simulink model "SF048A_TqLoa"  (R2013b)
settings: Solver=FixedStepDiscrete  SolverMode=SingleTasking  StartTime=0.0  StopTime=1  FixedStep=0.002  RelTol=1e-3
values from neighbouring files (symbols this model uses):
  ARCHGLBPRM_2MILLISEC_SEC_F32 = DataDict.Constant    [SF048A_TqLoa_DataDict.m]
  ARCHGLBPRM_PIOVER180_ULS_F32 = DataDict.Constant    [SF048A_TqLoa_DataDict.m]
  GRVYTLCON_MTRPERSECSQD_F32 = DataDict.Constant    [SF048A_TqLoa_DataDict.m]
  HWAUTHYMIN_ULS_F32 = DataDict.Constant    [SF048A_TqLoa_DataDict.m]
  MTRPERSECOVERKPH_MTRPERSECPERKPH_F32 = DataDict.Constant    [SF048A_TqLoa_DataDict.m]
  TqLoaDrvrTqNom = DataDict.Calibration    [SF048A_TqLoa_DataDict.m]
  TqLoaMotTqCmdLim = DataDict.Calibration    [SF048A_TqLoa_DataDict.m]
  TqLoaMotVelAndTqBasdScaFacMax = DataDict.Calibration    [SF048A_TqLoa_DataDict.m]
  TqLoaMotVelAndTqBasdScaFacMin = DataDict.Calibration    [SF048A_TqLoa_DataDict.m]
  TqLoaMotVelMgnThd = DataDict.Calibration    [SF048A_TqLoa_DataDict.m]
  TqLoaTqCmdMgnThd = DataDict.Calibration    [SF048A_TqLoa_DataDict.m]
  TqLoaVehSteerRat = DataDict.Calibration    [SF048A_TqLoa_DataDict.m]
  TqLoaVehUnderSteerGrdt = DataDict.Calibration    [SF048A_TqLoa_DataDict.m]
  TqLoaVehWhlBas = DataDict.Calibration    [SF048A_TqLoa_DataDict.m]
libraries: NxtrLim x8, FloatToFixd x5, FixdToFloat x4, LnrIntrpn x3, simulink x2, Fil x2, BilnrIntrpnCmnX x1
(part 1 of 2)
Description:
  | This function uses vehicle speed and HW position to generate a temporary position-based assist command.
  | This command is further scaled down based on vehicle speed, motor velocity and measured lateral
  | acceleration, to produce a final TLOA command.
settings Model: Creator=HZ69BY  LastModifiedBy=XZB1DB
settings Model: ModifiedHistory=|
  | Change Log:
  | Rev: 001
  | Date: 01Feb2015
  | Change Control #:
  | DRW:
  | Description:
  | - Initial Release
  | 
  | Rev: 002
  | Date: 05May2015
  | Change Request:  EA3#1132
  | Description:
  | - Removed Saturation from SF48A_TrqLOA_v002/TrqLOA/TrqLOA/Scaling/MtrVelBasedScaling/Torque-Velocity Based
  | - Added Saturation to SF48A_TrqLOA_v002/TrqLOA/TrqLOA/Scaling/VehicleSpeedBasedScaling
  | - Saturation limits set as constants from data dictionary
  | - Low-pass filter updated as per EA3 Simulink library (SF48A_TrqLOA_v002/TrqLOA/TrqLOA/Scaling/LatAccBasedScaling)
  | - Data Dictionary Changes:
  |    - t2_TrqLOA_DiffGainY_Uls_u1p15 name, table size, default value updated.
  |    - t_TrqLOA_DiffGainX_G_u2p14 default value updated
  |    - Changed range for k_TrqLOA_LimOutput_MtrNm_f32 & TrqLOACmd_MtrNm_f32
  |    - Added Constants d_TrqLOA_MinScale_Uls_f32 & d_TrqLOA_MaxScale_Uls_f32
  |    - Initial value of MotAgLoaMtgtnEn_Cnt_lgc changed to 0
  |    - Increased length/size of t_TrqLOA_X_Kph, t_TrqLOA_LatAccGain_Y_MtrNmpG, t_TrqLOA_TempTrqCmdSatYTbl_MtrNm
settings SolverCC: AutoInsertRateTranBlk=on  InsertRTBMode=Always
settings DataIOCC: LimitDataPoints=off  SaveFormat=Structure  ReturnWorkspaceOutputs=on
settings OptimizationCC: BlockReduction=off  InlineParams=on  ZeroExternalMemoryAtStartup=off  ZeroInternalMemoryAtStartup=off  OptimizeModelRefInitCode=on  LifeSpan=1
settings DebuggingCC: SignalInfNanChecking=error  SignalRangeChecking=warning  UnderspecifiedInitializationDetection=Simplified  SolverPrmCheckMsg=error  InheritedTsInSrcMsg=error  DiscreteInheritContinuousMsg=error  SingleTaskRateTransMsg=error  TasksWithSamePriorityMsg=error  SigSpecEnsureSampleTimeMsg=error  CheckMatrixSingularityMsg=error  ParameterUnderflowMsg=error  ParameterPrecisionLossMsg=error  ParameterTunabilityLossMsg=error  FixptConstUnderflowMsg=warning  FixptConstOverflowMsg=warning  VectorMatrixConversionMsg=error  SignalLabelMismatchMsg=error  UnconnectedInputMsg=error  UnconnectedOutputMsg=error  UnconnectedLineMsg=error  SFcnCompatibilityMsg=error  UniqueDataStoreMsg=warning  BusObjectLabelMismatch=error  RootOutportRequireBusObject=error  AssertControl=DisableAll  ModelReferenceIOMsg=error  ModelReferenceVersionMismatchMessage=warning  ModelReferenceIOMismatchMessage=error  ModelReferenceCSMismatchMessage=warning  ModelReferenceDataLoggingMessage=error  StateNameClashWarn=warning  StrictBusMsg=ErrorOnBusTreatedAsVector  NonBusSignalsTreatedAsBus=error  SFUnexpectedBacktrackingDiag=error  SFInvalidInputDataAccessInChartInitDiag=error  SFNoUnconditionalDefaultTransitionDiag=error  SFTransitionOutsideNaturalParentDiag=error  SFUnconditionalTransitionShadowingDiag=error  SFUndirectedBroadcastEventsDiag=error
settings ModelReferenceCC: ModelReferenceNumInstancesAllowed=Single
settings RTWCC: SystemTargetFile=autosar.tlc  GenCodeOnly=on  TemplateMakefile=ert_default_tmf  Description=AUTOSAR  GenerateReport=on  ProcessScript=autosar_make_rtw_hook  LaunchReport=on
settings CodeAppCC: GenerateComments=off  IgnoreCustomStorageClasses=off  CustomSymbolStrType=$N$R$M  CustomSymbolStrBlkIO=$N$M  SimulinkBlockComments=off
settings STFCustomTargetCC: ParMdlRefBuildCompliant=on  CompOptLevelCompliant=on  IncludeMdlTerminateFcn=off  CombineOutputUpdateFcns=on  SuppressErrorStatus=on  ERTFirstTimeCompliant=on  ERTCustomFileBanners=on  SupportNonFinite=off  SupportComplex=off  SupportContinuousTime=off  SupportNonInlinedSFcns=off  MATLABClassNameForMDSCustomization=Simulink.SoftwareTarget.ERTCustomization  AutosarCompliant=on  GRTInterface=off  SystemTargetFile=autosar.tlc
settings ERTTargetCC: CodeReplacementLibrary=ANSI_C  ConcurrentExecutionCompliant=off  IncludeMdlTerminateFcn=off  SuppressErrorStatus=on  SupportNonFinite=off  SupportComplex=off  ModelStepFunctionPrototypeControlCompliant=off  CPPClassGenCompliant=off  AutosarCompliant=on  InlinedParameterPlacement=NonHierarchical  ERTCustomFileTemplate=example_file_process.tlc  EnableUserReplacementTypes=on

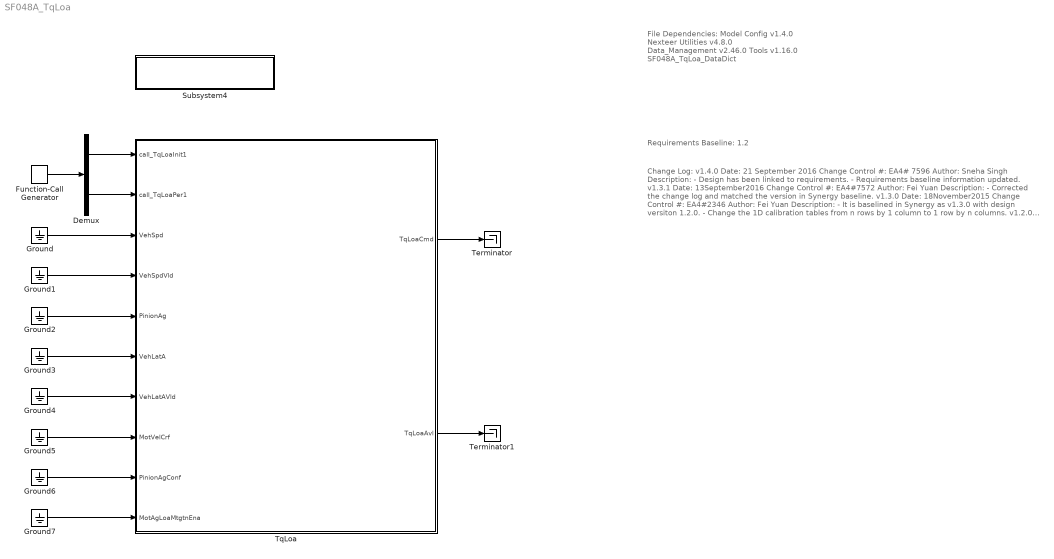
== system SF048A_TqLoa ==
  note: File Dependencies:
      |
      | Model Config v1.4.0
      | Nexteer Utilities v4.8.0
      | Data_Management v2.46.0
      | Tools v1.16.0
      | SF048A_TqLoa_DataDict
  note: Change Log:
      |
      | v1.4.0
      | Date: 21 September 2016
      | Change Control #: EA4# 7596
      | Author: Sneha Singh
      | Description:
      | - Design has been linked to requirements.
      | - Requirements baseline information updated.
      |
      | v1.3.1
      | Date: 13September2016
      | Change Control #: EA4#7572
      | Author: Fei Yuan
      | Description:
      | - Corrected the change log and matched the version in Synergy baseline.
      |
      | v1.3.0
      | Date: 18November2015
      | Change Control #: EA4#2346
      | Author: Fei Yuan
      | Description:
      | - It is baselined in Synergy as v1.3.0 with design versiton 1.2.0.
      | - Change the 1D calibration tables from n rows by 1 column to 1 row by n
      |   columns.
      |
      | v1.2.0
      | Date: 01September2015
      | Change Control #: EA4#1010
      | DRW: P.Lefler
      | Description:
      | - It is baselined in Synergy as v1.2.0 with design version 1.1.0.
      |
      |
      | v1.1.0
      | Date: 01September2015
      | Change Control #: EA4#1010
      | DRW: P. Lefler
      | Description:
      | - Fixed reversed order of constants in static limit blocks.
      | - Removed extra write to a display variable.
      | - Changed inputs from HwAg and HwAuthy to PinionAgConf and PinionAg
      |
      |
      | v1.0.0
      | Date: 30July2015
      | Change Control #: EA4#1010
      | DRW: P. Lefler
      | Description:
      | - Initial Release
  note: Requirements Baseline: 1.2
  Demux : Demux  Outputs=2
  Function-Call Generator : simulink/Ports & Subsystems/Function-Call Generator  sample_time=0.002  numberOfIterations=1
  Ground{,1..7} (8 alike) : Ground
  Subsystem4 : Subsystem  Description=|  mask(Copyright Information){none=on}
      | Copyright info block.                                               
      |                                                                     
      | Place copyright information at the top of every subsystem in design.
      mask prompts: none "No parameters"
      mask help: Place copyright information at the top of every subsystem in design.
      mask Display:
      | NxtrConf = 'Nexteer Confidential';
      | 
      | sys = bdroot; %handle for the current model ("system")
      | first = get_param(sys,'Created');
      | first = first(end-3:end);  %year is last four digits
      | 
      | last = get_param(sys,'LastModifiedDate');
      | if isempty(last)
      |     last = datestr(now,'yyyy');
      | else
      |     last = last(end-3:end);
      | end
      | 
      | if strcmp(first,last)
      |     fprintf('%s\nCopyright  %s Nexteer',NxtrConf,first);
      | else
      |     fprintf('%s\n%s%s-%s Nexteer',NxtrConf,char(169),first,last);
      | end
  Terminator : Terminator
  Terminator1 : Terminator
  TqLoa : Subsystem
  wires:
  TqLoa/1(TqLoaCmd) -> Terminator/1
  TqLoa/2(TqLoaAvl) -> Terminator1/1
  Ground7/1 -> TqLoa/10(MotAgLoaMtgtnEna)
  Ground6/1 -> TqLoa/9(PinionAgConf)
  Demux/1 -> TqLoa/1(call_TqLoaInit1)
  Demux/2 -> TqLoa/2(call_TqLoaPer1)
  Function-Call Generator/1 -> Demux/1
  Ground4/1 -> TqLoa/7(VehLatAVld)
  Ground2/1 -> TqLoa/5(PinionAg)
  Ground/1 -> TqLoa/3(VehSpd)
  Ground1/1 -> TqLoa/4(VehSpdVld)
  Ground3/1 -> TqLoa/6(VehLatA)
  Ground5/1 -> TqLoa/8(MotVelCrf)

== system SF048A_TqLoa/Subsystem4 ==

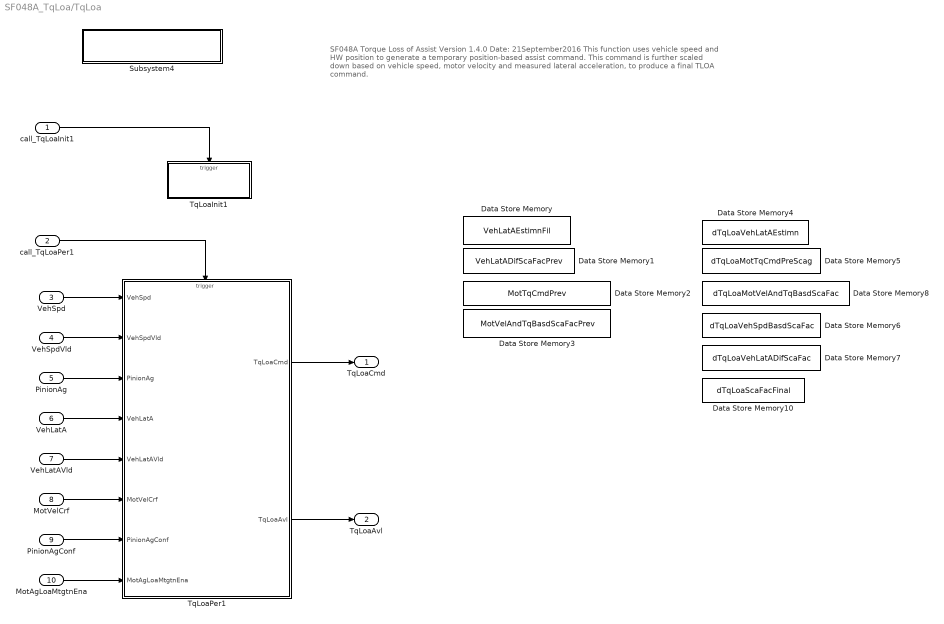
== system SF048A_TqLoa/TqLoa ==
  note: SF048A Torque Loss of Assist
      | Version 1.4.0			Date: 21September2016
      | This function uses vehicle speed and HW position to generate a temporary position-based assist command.
      | This command is further scaled down based on vehicle speed, motor velocity and measured lateral
      | acceleration, to produce a final TLOA command.
  call_TqLoaInit1 : Inport
  call_TqLoaPer1 : Inport  Port=2
  VehSpd : Inport  RequirementInfo="{'linktype_rmi_doors' '0000ba57 (/E-STEER Core/SubSystem Specifications/Application Functions/SF048A Torque Sensor LOA)' '#SF048A_6' 'true' 'REQ:  SF048A_6' '' } %GIDa_a3883147_9782_4e4b_8e21_1803a965b4c0"  Port=3
  VehSpdVld : Inport  RequirementInfo="{'linktype_rmi_doors' '0000ba57 (/E-STEER Core/SubSystem Specifications/Application Functions/SF048A Torque Sensor LOA)' '#SF048A_6' 'true' 'REQ:  SF048A_6' '' } %GIDa_02708a8b_8017_404a_990b_357237815eff"  Port=4
  PinionAg : Inport  RequirementInfo="{'linktype_rmi_doors' '0000ba57 (/E-STEER Core/SubSystem Specifications/Application Functions/SF048A Torque Sensor LOA)' '#SF048A_7' 'true' 'REQ:  SF048A_7' '' } %GIDa_9e569ae1_e816_4a3a_b96f_f5710bee6e9e"  Port=5
  VehLatA : Inport  RequirementInfo="{'linktype_rmi_doors' '0000ba57 (/E-STEER Core/SubSystem Specifications/Application Functions/SF048A Torque Sensor LOA)' '#SF048A_40' 'true' 'REQ:  SF048A_40' '' } %GIDa_13b7e215_ca06_42b4_96ce_87e09b7122fe"  Port=6
  VehLatAVld : Inport  RequirementInfo="{'linktype_rmi_doors' '0000ba57 (/E-STEER Core/SubSystem Specifications/Application Functions/SF048A Torque Sensor LOA)' '#SF048A_41' 'true' 'REQ:  SF048A_41' '' } %GIDa_2dd0dbe9_8486_4322_8285_2c1192106a5d"  Port=7
  MotVelCrf : Inport  RequirementInfo="{'linktype_rmi_doors' '0000ba57 (/E-STEER Core/SubSystem Specifications/Application Functions/SF048A Torque Sensor LOA)' '#SF048A_42' 'true' 'REQ:  SF048A_42' '' } %GIDa_5a1973eb_7739_48b8_9cc6_d351e8423a12"  Port=8
  PinionAgConf : Inport  RequirementInfo="{'linktype_rmi_doors' '0000ba57 (/E-STEER Core/SubSystem Specifications/Application Functions/SF048A Torque Sensor LOA)' '#SF048A_8' 'true' 'REQ:  SF048A_8' '' } %GIDa_aa7a9f1f_eb7f_4301_85f9_898c0a77cdeb"  Port=9
  MotAgLoaMtgtnEna : Inport  RequirementInfo="{'linktype_rmi_doors' '0000ba57 (/E-STEER Core/SubSystem Specifications/Application Functions/SF048A Torque Sensor LOA)' '#SF048A_43' 'true' 'REQ:  SF048A_43' '' } %GIDa_2270dc32_128a_4873_b3c1_ebcb33cb1a8b"  Port=10
  Data Store Memory : DataStoreMemory  DataStoreName=VehLatAEstimnFil  InitialValue=[]  StateMustResolveToSignalObject=on
  Data Store Memory1 : DataStoreMemory  DataStoreName=VehLatADifScaFacPrev  StateMustResolveToSignalObject=on
  Data Store Memory10 : DataStoreMemory  DataStoreName=dTqLoaScaFacFinal  ReadBeforeWriteMsg=warning  WriteAfterWriteMsg=warning  WriteAfterReadMsg=warning  StateMustResolveToSignalObject=on
  Data Store Memory2 : DataStoreMemory  DataStoreName=MotTqCmdPrev  StateMustResolveToSignalObject=on
  Data Store Memory3 : DataStoreMemory  DataStoreName=MotVelAndTqBasdScaFacPrev  StateMustResolveToSignalObject=on
  Data Store Memory4 : DataStoreMemory  DataStoreName=dTqLoaVehLatAEstimn  ReadBeforeWriteMsg=warning  WriteAfterWriteMsg=warning  WriteAfterReadMsg=warning  StateMustResolveToSignalObject=on
  Data Store Memory5 : DataStoreMemory  DataStoreName=dTqLoaMotTqCmdPreScag  ReadBeforeWriteMsg=warning  WriteAfterWriteMsg=warning  WriteAfterReadMsg=warning  StateMustResolveToSignalObject=on
  Data Store Memory6 : DataStoreMemory  DataStoreName=dTqLoaVehSpdBasdScaFac  ReadBeforeWriteMsg=warning  WriteAfterWriteMsg=warning  WriteAfterReadMsg=warning  StateMustResolveToSignalObject=on
  Data Store Memory7 : DataStoreMemory  DataStoreName=dTqLoaVehLatADifScaFac  ReadBeforeWriteMsg=warning  WriteAfterWriteMsg=warning  WriteAfterReadMsg=warning  StateMustResolveToSignalObject=on
  Data Store Memory8 : DataStoreMemory  DataStoreName=dTqLoaMotVelAndTqBasdScaFac  ReadBeforeWriteMsg=warning  WriteAfterWriteMsg=warning  WriteAfterReadMsg=warning  StateMustResolveToSignalObject=on
  Subsystem4 : Subsystem  Description=|  mask(Copyright Information){none=on}
      | Copyright info block.                                               
      |                                                                     
      | Place copyright information at the top of every subsystem in design.
      mask prompts: none "No parameters"
      mask help: Place copyright information at the top of every subsystem in design.
      mask Display:
      | NxtrConf = 'Nexteer Confidential';
      | 
      | sys = bdroot; %handle for the current model ("system")
      | first = get_param(sys,'Created');
      | first = first(end-3:end);  %year is last four digits
      | 
      | last = get_param(sys,'LastModifiedDate');
      | if isempty(last)
      |     last = datestr(now,'yyyy');
      | else
      |     last = last(end-3:end);
      | end
      | 
      | if strcmp(first,last)
      |     fprintf('%s\nCopyright  %s Nexteer',NxtrConf,first);
      | else
      |     fprintf('%s\n%s%s-%s Nexteer',NxtrConf,char(169),first,last);
      | end
  TqLoaInit1 : Subsystem
  TqLoaPer1 : Subsystem
  TqLoaCmd : Outport  RequirementInfo="{'linktype_rmi_doors' '0000ba57 (/E-STEER Core/SubSystem Specifications/Application Functions/SF048A Torque Sensor LOA)' '#SF048A_10' 'true' 'REQ:  SF048A_10' '' } %GIDa_df82e166_2ee0_4c30_8d9b_00a7e29d6193"
  TqLoaAvl : Outport  RequirementInfo="{'linktype_rmi_doors' '0000ba57 (/E-STEER Core/SubSystem Specifications/Application Functions/SF048A Torque Sensor LOA)' '#SF048A_44' 'true' 'REQ:  SF048A_44' '' } %GIDa_bf8a2443_6d8b_4475_a369_59109990c7ac"  Port=2
  wires:
  MotAgLoaMtgtnEna/1 -> TqLoaPer1/8(MotAgLoaMtgtnEna)
  MotVelCrf/1 -> TqLoaPer1/6(MotVelCrf)
  VehLatAVld/1 -> TqLoaPer1/5(VehLatAVld)
  PinionAg/1 -> TqLoaPer1/3(PinionAg)
  VehSpdVld/1 -> TqLoaPer1/2(VehSpdVld)
  VehLatA/1 -> TqLoaPer1/4(VehLatA)
  PinionAgConf/1 -> TqLoaPer1/7(PinionAgConf)
  VehSpd/1 -> TqLoaPer1/1(VehSpd)
  TqLoaPer1/1(TqLoaCmd) -> TqLoaCmd/1
  TqLoaPer1/2(TqLoaAvl) -> TqLoaAvl/1
  call_TqLoaPer1/1 -> TqLoaPer1/Trigger
  call_TqLoaInit1/1 -> TqLoaInit1/Trigger

== system SF048A_TqLoa/TqLoa/Subsystem4 ==

== system SF048A_TqLoa/TqLoa/TqLoaInit1 ==
  Function : TriggerPort  TriggerType=function-call  PortDimensions=1
  FilLpInit : Fil/FilLpInit  Ic=0  Ts=ARCHGLBPRM_2MILLISEC_SEC_F32  Freq=TqLoaVehLatAEstimnFilFrq  StVar=VehLatAEstimnFil
  Subsystem4 : Subsystem  Description=|  mask(Copyright Information){none=on}
      | Copyright info block.                                               
      |                                                                     
      | Place copyright information at the top of every subsystem in design.
      mask prompts: none "No parameters"
      mask help: Place copyright information at the top of every subsystem in design.
      mask Display:
      | NxtrConf = 'Nexteer Confidential';
      | 
      | sys = bdroot; %handle for the current model ("system")
      | first = get_param(sys,'Created');
      | first = first(end-3:end);  %year is last four digits
      | 
      | last = get_param(sys,'LastModifiedDate');
      | if isempty(last)
      |     last = datestr(now,'yyyy');
      | else
      |     last = last(end-3:end);
      | end
      | 
      | if strcmp(first,last)
      |     fprintf('%s\nCopyright  %s Nexteer',NxtrConf,first);
      | else
      |     fprintf('%s\n%s%s-%s Nexteer',NxtrConf,char(169),first,last);
      | end

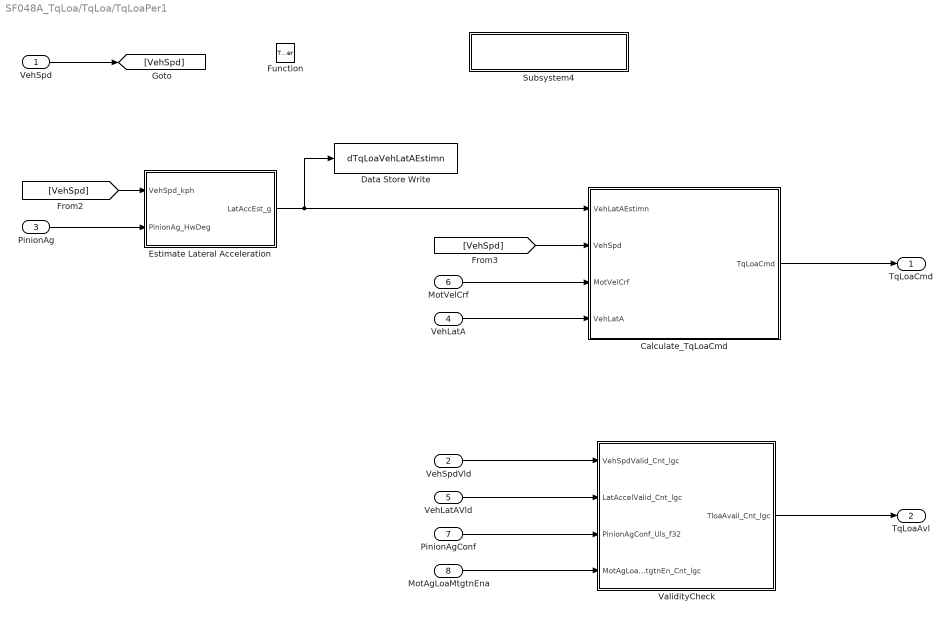
== system SF048A_TqLoa/TqLoa/TqLoaPer1 ==
  VehSpd : Inport
  VehSpdVld : Inport  Port=2
  PinionAg : Inport  Port=3
  VehLatA : Inport  Port=4
  VehLatAVld : Inport  Port=5
  MotVelCrf : Inport  Port=6
  PinionAgConf : Inport  Port=7
  MotAgLoaMtgtnEna : Inport  Port=8
  Function : TriggerPort  TriggerType=function-call  PortDimensions=1
  Calculate_TqLoaCmd : Subsystem
  Data Store Write : DataStoreWrite  DataStoreName=dTqLoaVehLatAEstimn
  Estimate Lateral Acceleration : Subsystem  RequirementInfo="{'linktype_rmi_doors' '0000ba57 (/E-STEER Core/SubSystem Specifications/Application Functions/SF048A Torque Sensor LOA)' '#SF048A_57' 'true' 'REQ:  SF048A_57' '' } %GIDa_a7e7015c_6445_44b2_86c9_655a6d6cfbb8"
  Subsystem4 : Subsystem  Description=|  mask(Copyright Information){none=on}
      | Copyright info block.                                               
      |                                                                     
      | Place copyright information at the top of every subsystem in design.
      mask prompts: none "No parameters"
      mask help: Place copyright information at the top of every subsystem in design.
      mask Display:
      | NxtrConf = 'Nexteer Confidential';
      | 
      | sys = bdroot; %handle for the current model ("system")
      | first = get_param(sys,'Created');
      | first = first(end-3:end);  %year is last four digits
      | 
      | last = get_param(sys,'LastModifiedDate');
      | if isempty(last)
      |     last = datestr(now,'yyyy');
      | else
      |     last = last(end-3:end);
      | end
      | 
      | if strcmp(first,last)
      |     fprintf('%s\nCopyright  %s Nexteer',NxtrConf,first);
      | else
      |     fprintf('%s\n%s%s-%s Nexteer',NxtrConf,char(169),first,last);
      | end
  ValidityCheck : Subsystem
  TqLoaCmd : Outport
  TqLoaAvl : Outport  Port=2
  wires:
  Estimate Lateral Acceleration/1(LatAccEst_g) -> Data Store Write/1, Calculate_TqLoaCmd/1(VehLatAEstimn)
  [VehSpd] -> Estimate Lateral Acceleration/1(VehSpd_kph)
  ValidityCheck/1(TloaAvail_Cnt_lgc) -> TqLoaAvl/1
  VehSpd/1 -> [VehSpd]
  VehSpdVld/1 -> ValidityCheck/1(VehSpdValid_Cnt_lgc)
  MotAgLoaMtgtnEna/1 -> ValidityCheck/4(MotAgLoaMtgtnEn_Cnt_lgc)
  PinionAgConf/1 -> ValidityCheck/3(PinionAgConf_Uls_f32)
  VehLatAVld/1 -> ValidityCheck/2(LatAccelValid_Cnt_lgc)
  PinionAg/1 -> Estimate Lateral Acceleration/2(PinionAg_HwDeg)
  [VehSpd] -> Calculate_TqLoaCmd/2(VehSpd)
  MotVelCrf/1 -> Calculate_TqLoaCmd/3(MotVelCrf)
  VehLatA/1 -> Calculate_TqLoaCmd/4(VehLatA)
  Calculate_TqLoaCmd/1(TqLoaCmd) -> TqLoaCmd/1

== system SF048A_TqLoa/TqLoa/TqLoaInit1/Subsystem4 ==

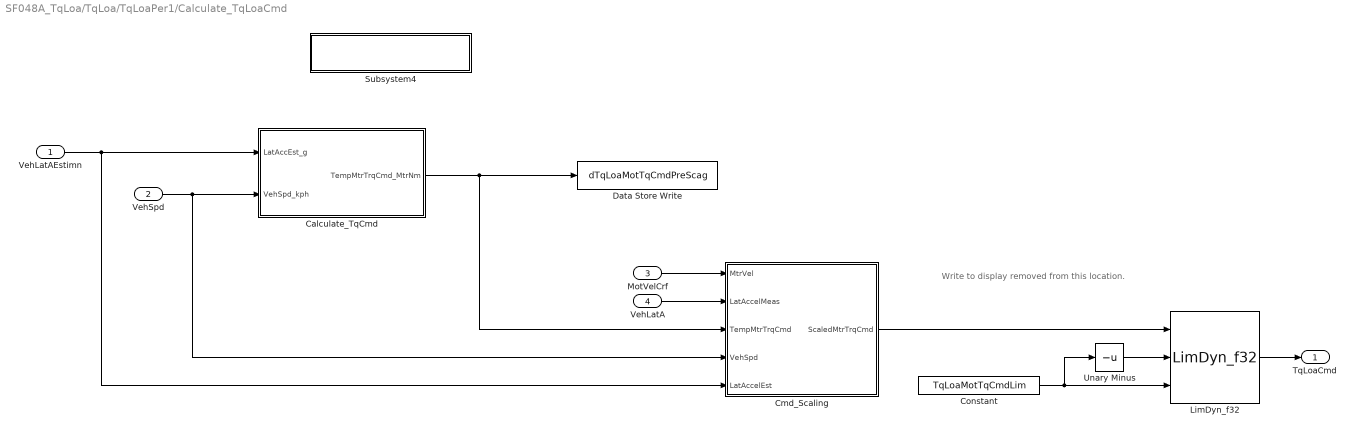
== system SF048A_TqLoa/TqLoa/TqLoaPer1/Calculate_TqLoaCmd ==
  note: Write to display removed from this location.
  VehLatAEstimn : Inport
  VehSpd : Inport  Port=2
  MotVelCrf : Inport  Port=3
  VehLatA : Inport  Port=4
  Calculate_TqCmd : Subsystem
  Cmd_Scaling : Subsystem
  Constant : Constant  RequirementInfo="{'linktype_rmi_doors' '0000ba57 (/E-STEER Core/SubSystem Specifications/Application Functions/SF048A Torque Sensor LOA)' '#SF048A_83' 'true' 'REQ:  SF048A_83' '' } %GIDa_345a0c70_3a23_42e4_82c5_17cc6df77ff3"  Value=TqLoaMotTqCmdLim
  Data Store Write : DataStoreWrite  DataStoreName=dTqLoaMotTqCmdPreScag
  LimDyn_f32 : NxtrLim/LimDyn_f32  RequirementInfo="{'linktype_rmi_doors' '0000ba57 (/E-STEER Core/SubSystem Specifications/Application Functions/SF048A Torque Sensor LOA)' '#SF048A_83' 'true' 'REQ:  SF048A_83' '' } %GIDa_4f3c0232_1e79_429d_a984_0b97885bf63a"
  Subsystem4 : Subsystem  Description=|  mask(Copyright Information){none=on}
      | Copyright info block.                                               
      |                                                                     
      | Place copyright information at the top of every subsystem in design.
      mask prompts: none "No parameters"
      mask help: Place copyright information at the top of every subsystem in design.
      mask Display:
      | NxtrConf = 'Nexteer Confidential';
      | 
      | sys = bdroot; %handle for the current model ("system")
      | first = get_param(sys,'Created');
      | first = first(end-3:end);  %year is last four digits
      | 
      | last = get_param(sys,'LastModifiedDate');
      | if isempty(last)
      |     last = datestr(now,'yyyy');
      | else
      |     last = last(end-3:end);
      | end
      | 
      | if strcmp(first,last)
      |     fprintf('%s\nCopyright  %s Nexteer',NxtrConf,first);
      | else
      |     fprintf('%s\n%s%s-%s Nexteer',NxtrConf,char(169),first,last);
      | end
  Unary Minus : UnaryMinus  RequirementInfo="{'linktype_rmi_doors' '0000ba57 (/E-STEER Core/SubSystem Specifications/Application Functions/SF048A Torque Sensor LOA)' '#SF048A_83' 'true' 'REQ:  SF048A_83' '' } %GIDa_18624763_2337_4b9b_9e4e_a1ba6e2cdcf8"
  TqLoaCmd : Outport
  wires:
  VehLatAEstimn/1 -> Cmd_Scaling/5(LatAccelEst), Calculate_TqCmd/1(LatAccEst_g)
  VehSpd/1 -> Cmd_Scaling/4(VehSpd), Calculate_TqCmd/2(VehSpd_kph)
  LimDyn_f32/1 -> TqLoaCmd/1
  Calculate_TqCmd/1(TempMtrTrqCmd_MtrNm) -> Cmd_Scaling/3(TempMtrTrqCmd), Data Store Write/1
  VehLatA/1 -> Cmd_Scaling/2(LatAccelMeas)
  Cmd_Scaling/1(ScaledMtrTrqCmd) -> LimDyn_f32/1
  MotVelCrf/1 -> Cmd_Scaling/1(MtrVel)
  Constant/1 -> LimDyn_f32/3, Unary Minus/1
  Unary Minus/1 -> LimDyn_f32/2

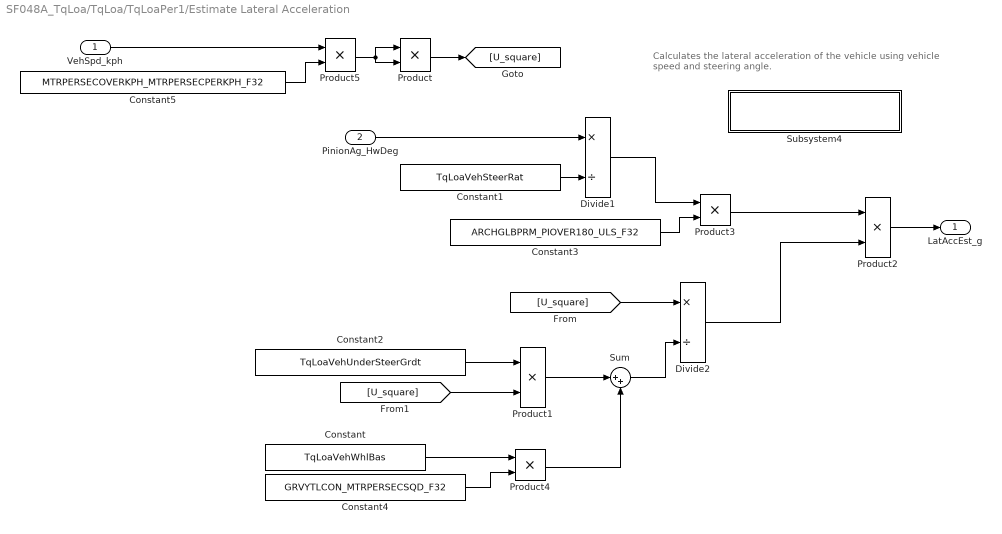
== system SF048A_TqLoa/TqLoa/TqLoaPer1/Estimate Lateral Acceleration ==
  note: Calculates the lateral acceleration of the vehicle
      | using vehicle speed and steering angle.
  VehSpd_kph : Inport
  PinionAg_HwDeg : Inport  Port=2
  Constant : Constant  Value=TqLoaVehWhlBas
  Constant1 : Constant  Value=TqLoaVehSteerRat
  Constant2 : Constant  Value=TqLoaVehUnderSteerGrdt
  Constant3 : Constant  Value=ARCHGLBPRM_PIOVER180_ULS_F32
  Constant4 : Constant  Value=GRVYTLCON_MTRPERSECSQD_F32
  Constant5 : Constant  Value=MTRPERSECOVERKPH_MTRPERSECPERKPH_F32
  Divide1 : Product  Inputs=*/
  Divide2 : Product  Inputs=*/
  Product{,1..2,5} (4 alike) : Product  RndMeth=Zero
  Product3 : Product
  Product4 : Product
  Subsystem4 : Subsystem  Description=|  mask(Copyright Information){none=on}
      | Copyright info block.                                               
      |                                                                     
      | Place copyright information at the top of every subsystem in design.
      mask prompts: none "No parameters"
      mask help: Place copyright information at the top of every subsystem in design.
      mask Display:
      | NxtrConf = 'Nexteer Confidential';
      | 
      | sys = bdroot; %handle for the current model ("system")
      | first = get_param(sys,'Created');
      | first = first(end-3:end);  %year is last four digits
      | 
      | last = get_param(sys,'LastModifiedDate');
      | if isempty(last)
      |     last = datestr(now,'yyyy');
      | else
      |     last = last(end-3:end);
      | end
      | 
      | if strcmp(first,last)
      |     fprintf('%s\nCopyright  %s Nexteer',NxtrConf,first);
      | else
      |     fprintf('%s\n%s%s-%s Nexteer',NxtrConf,char(169),first,last);
      | end
  Sum : Sum  Inputs=|++
  LatAccEst_g : Outport
  wires:
  Product3/1 -> Product2/1
  Product2/1 -> LatAccEst_g/1
  Divide2/1 -> Product2/2
  Divide1/1 -> Product3/1
  Sum/1 -> Divide2/2
  Product4/1 -> Sum/2
  Product1/1 -> Sum/1
  [U_square] -> Product1/2
  Constant2/1 -> Product1/1
  [U_square] -> Divide2/1
  Product/1 -> [U_square]
  Constant/1 -> Product4/1
  Constant1/1 -> Divide1/2
  PinionAg_HwDeg/1 -> Divide1/1
  Constant3/1 -> Product3/2
  Constant4/1 -> Product4/2
  Constant5/1 -> Product5/2
  VehSpd_kph/1 -> Product5/1
  Product5/1 -> Product/2, Product/1

== system SF048A_TqLoa/TqLoa/TqLoaPer1/Subsystem4 ==

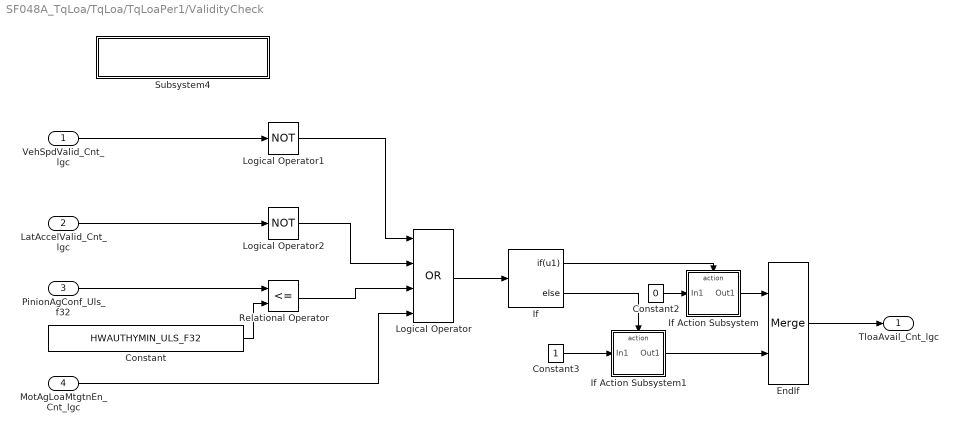
== system SF048A_TqLoa/TqLoa/TqLoaPer1/ValidityCheck ==
  VehSpdValid_Cnt_lgc : Inport  RequirementInfo="{'linktype_rmi_doors' '0000ba57 (/E-STEER Core/SubSystem Specifications/Application Functions/SF048A Torque Sensor LOA)' '#SF048A_85' 'true' 'REQ:  SF048A_85' '' ; 'linktype_rmi_doors' '0000ba57 (/E-STEER Core/SubSystem Specifications/Application Functions/SF048A Torque Sensor LOA)' '#SF048A_86' 'true' 'REQ:  SF048A_86' '' } %GIDa_744cf0d6_c0a0_4492_95a3_0b941d8f8dbf"
  LatAccelValid_Cnt_lgc : Inport  RequirementInfo="{'linktype_rmi_doors' '0000ba57 (/E-STEER Core/SubSystem Specifications/Application Functions/SF048A Torque Sensor LOA)' '#SF048A_85' 'true' 'REQ:  SF048A_85' '' ; 'linktype_rmi_doors' '0000ba57 (/E-STEER Core/SubSystem Specifications/Application Functions/SF048A Torque Sensor LOA)' '#SF048A_86' 'true' 'REQ:  SF048A_86' '' } %GIDa_bb8d3005_464a_48b6_aad8_efd47d22c1cc"  Port=2
  PinionAgConf_Uls_f32 : Inport  RequirementInfo="{'linktype_rmi_doors' '0000ba57 (/E-STEER Core/SubSystem Specifications/Application Functions/SF048A Torque Sensor LOA)' '#SF048A_85' 'true' 'REQ:  SF048A_85' '' ; 'linktype_rmi_doors' '0000ba57 (/E-STEER Core/SubSystem Specifications/Application Functions/SF048A Torque Sensor LOA)' '#SF048A_86' 'true' 'REQ:  SF048A_86' '' } %GIDa_e4b1b9b4_d11d_4319_bb06_a6fcfe27e8a2"  Port=3
  MotAgLoaMtgtnEn_Cnt_lgc : Inport  RequirementInfo="{'linktype_rmi_doors' '0000ba57 (/E-STEER Core/SubSystem Specifications/Application Functions/SF048A Torque Sensor LOA)' '#SF048A_85' 'true' 'REQ:  SF048A_85' '' ; 'linktype_rmi_doors' '0000ba57 (/E-STEER Core/SubSystem Specifications/Application Functions/SF048A Torque Sensor LOA)' '#SF048A_86' 'true' 'REQ:  SF048A_86' '' } %GIDa_734fd1c1_7087_4130_a0ab_1fdc662302d6"  Port=4
  Constant : Constant  RequirementInfo="{'linktype_rmi_doors' '0000ba57 (/E-STEER Core/SubSystem Specifications/Application Functions/SF048A Torque Sensor LOA)' '#SF048A_85' 'true' 'REQ:  SF048A_85' '' ; 'linktype_rmi_doors' '0000ba57 (/E-STEER Core/SubSystem Specifications/Application Functions/SF048A Torque Sensor LOA)' '#SF048A_86' 'true' 'REQ:  SF048A_86' '' } %GIDa_012c227c_6d65_42a4_84b8_e4880d3507eb"  Value=HWAUTHYMIN_ULS_F32
  Constant2 : Constant  RequirementInfo="{'linktype_rmi_doors' '0000ba57 (/E-STEER Core/SubSystem Specifications/Application Functions/SF048A Torque Sensor LOA)' '#SF048A_85' 'true' 'REQ:  SF048A_85' '' } %GIDa_16f623ce_c0da_4cf8_901d_ae48ec2ceeff"  Value=0  OutDataTypeStr=boolean
      settings: AttributesFormatString=FALSE
  Constant3 : Constant  RequirementInfo="{'linktype_rmi_doors' '0000ba57 (/E-STEER Core/SubSystem Specifications/Application Functions/SF048A Torque Sensor LOA)' '#SF048A_86' 'true' 'REQ:  SF048A_86' '' } %GIDa_f114bc94_db30_4bf2_8bb1_6377d035bafc"  OutDataTypeStr=boolean
      settings: AttributesFormatString=TRUE
  EndIf : Merge
  If : If  RequirementInfo="{'linktype_rmi_doors' '0000ba57 (/E-STEER Core/SubSystem Specifications/Application Functions/SF048A Torque Sensor LOA)' '#SF048A_85' 'true' 'REQ:  SF048A_85' '' ; 'linktype_rmi_doors' '0000ba57 (/E-STEER Core/SubSystem Specifications/Application Functions/SF048A Torque Sensor LOA)' '#SF048A_86' 'true' 'REQ:  SF048A_86' '' } %GIDa_e67fc9fe_2b7e_41d8_b7a9_54eec1f7c32c"  IfExpression=u1
  If Action Subsystem : Subsystem  RequirementInfo="{'linktype_rmi_doors' '0000ba57 (/E-STEER Core/SubSystem Specifications/Application Functions/SF048A Torque Sensor LOA)' '#SF048A_85' 'true' 'REQ:  SF048A_85' '' } %GIDa_975dfdca_8abf_4b70_8e6d_8e1ed5e75d74"  TreatAsAtomicUnit=on
  If Action Subsystem1 : Subsystem  RequirementInfo="{'linktype_rmi_doors' '0000ba57 (/E-STEER Core/SubSystem Specifications/Application Functions/SF048A Torque Sensor LOA)' '#SF048A_86' 'true' 'REQ:  SF048A_86' '' } %GIDa_b968aece_01be_43c2_ae18_bc0b9cea340b"  TreatAsAtomicUnit=on
  Logical Operator : Logic  RequirementInfo="{'linktype_rmi_doors' '0000ba57 (/E-STEER Core/SubSystem Specifications/Application Functions/SF048A Torque Sensor LOA)' '#SF048A_85' 'true' 'REQ:  SF048A_85' '' ; 'linktype_rmi_doors' '0000ba57 (/E-STEER Core/SubSystem Specifications/Application Functions/SF048A Torque Sensor LOA)' '#SF048A_86' 'true' 'REQ:  SF048A_86' '' } %GIDa_8bcd2a43_661a_407c_a131_0c0b3880a8ea"  Operator=OR  Inputs=4  AllPortsSameDT=off  OutDataTypeStr=boolean
  Logical Operator1 : Logic  RequirementInfo="{'linktype_rmi_doors' '0000ba57 (/E-STEER Core/SubSystem Specifications/Application Functions/SF048A Torque Sensor LOA)' '#SF048A_85' 'true' 'REQ:  SF048A_85' '' ; 'linktype_rmi_doors' '0000ba57 (/E-STEER Core/SubSystem Specifications/Application Functions/SF048A Torque Sensor LOA)' '#SF048A_86' 'true' 'REQ:  SF048A_86' '' } %GIDa_cf3a1ce6_7543_4fdc_9297_b1288c4d4b73"  Operator=NOT  AllPortsSameDT=off  OutDataTypeStr=boolean
  Logical Operator2 : Logic  RequirementInfo="{'linktype_rmi_doors' '0000ba57 (/E-STEER Core/SubSystem Specifications/Application Functions/SF048A Torque Sensor LOA)' '#SF048A_85' 'true' 'REQ:  SF048A_85' '' ; 'linktype_rmi_doors' '0000ba57 (/E-STEER Core/SubSystem Specifications/Application Functions/SF048A Torque Sensor LOA)' '#SF048A_86' 'true' 'REQ:  SF048A_86' '' } %GIDa_aa900443_a7fc_40ed_9c53_b4db7117c40e"  Operator=NOT  AllPortsSameDT=off  OutDataTypeStr=boolean
  Relational Operator : RelationalOperator  RequirementInfo="{'linktype_rmi_doors' '0000ba57 (/E-STEER Core/SubSystem Specifications/Application Functions/SF048A Torque Sensor LOA)' '#SF048A_85' 'true' 'REQ:  SF048A_85' '' ; 'linktype_rmi_doors' '0000ba57 (/E-STEER Core/SubSystem Specifications/Application Functions/SF048A Torque Sensor LOA)' '#SF048A_86' 'true' 'REQ:  SF048A_86' '' } %GIDa_00e96ab6_a16b_4f1b_aa0d_b2246bad26d6"  Operator=<=  OutDataTypeStr=boolean
  Subsystem4 : Subsystem  Description=|  mask(Copyright Information){none=on}
      | Copyright info block.                                               
      |                                                                     
      | Place copyright information at the top of every subsystem in design.
      mask prompts: none "No parameters"
      mask help: Place copyright information at the top of every subsystem in design.
      mask Display:
      | NxtrConf = 'Nexteer Confidential';
      | 
      | sys = bdroot; %handle for the current model ("system")
      | first = get_param(sys,'Created');
      | first = first(end-3:end);  %year is last four digits
      | 
      | last = get_param(sys,'LastModifiedDate');
      | if isempty(last)
      |     last = datestr(now,'yyyy');
      | else
      |     last = last(end-3:end);
      | end
      | 
      | if strcmp(first,last)
      |     fprintf('%s\nCopyright  %s Nexteer',NxtrConf,first);
      | else
      |     fprintf('%s\n%s%s-%s Nexteer',NxtrConf,char(169),first,last);
      | end
  TloaAvail_Cnt_lgc : Outport
  wires:
  Logical Operator/1 -> If/1
  PinionAgConf_Uls_f32/1 -> Relational Operator/1
  VehSpdValid_Cnt_lgc/1 -> Logical Operator1/1
  LatAccelValid_Cnt_lgc/1 -> Logical Operator2/1
  If/1 -> If Action Subsystem/Action
  If Action Subsystem/1(Out1) -> EndIf/1
  Constant2/1 -> If Action Subsystem/1(In1)
  If/2 -> If Action Subsystem1/Action
  EndIf/1 -> TloaAvail_Cnt_lgc/1
  MotAgLoaMtgtnEn_Cnt_lgc/1 -> Logical Operator/4
  Logical Operator1/1 -> Logical Operator/1
  Logical Operator2/1 -> Logical Operator/2
  Relational Operator/1 -> Logical Operator/3
  Constant3/1 -> If Action Subsystem1/1(In1)
  If Action Subsystem1/1(Out1) -> EndIf/2
  Constant/1 -> Relational Operator/2

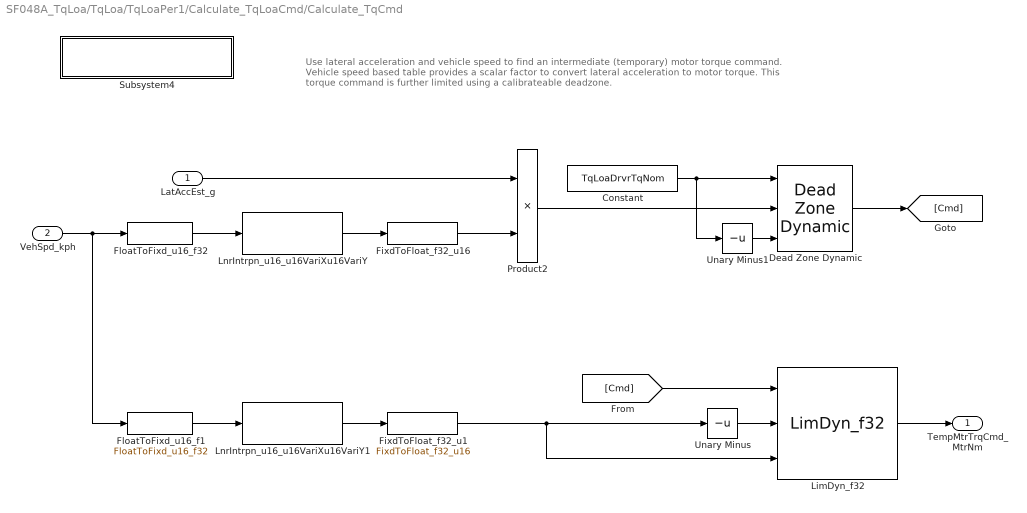
== system SF048A_TqLoa/TqLoa/TqLoaPer1/Calculate_TqLoaCmd/Calculate_TqCmd ==
  note: Use lateral acceleration and vehicle speed to find an intermediate (temporary) motor torque command.
      | Vehicle speed based table provides a scalar factor to convert lateral acceleration to motor torque. This
      | torque command is further limited using a calibrateable deadzone.
  LatAccEst_g : Inport  RequirementInfo="{'linktype_rmi_doors' '0000ba57 (/E-STEER Core/SubSystem Specifications/Application Functions/SF048A Torque Sensor LOA)' '#SF048A_60' 'true' 'REQ:  SF048A_60' '' } %GIDa_ae829d5b_30e1_47fc_872c_8347a4fcb1ed"
  VehSpd_kph : Inport  RequirementInfo="{'linktype_rmi_doors' '0000ba57 (/E-STEER Core/SubSystem Specifications/Application Functions/SF048A Torque Sensor LOA)' '#SF048A_60' 'true' 'REQ:  SF048A_60' '' } %GIDa_d3e87a5d_77d3_47cf_95da_3c1013e6a80e"  Port=2
  Constant : Constant  RequirementInfo="{'linktype_rmi_doors' '0000ba57 (/E-STEER Core/SubSystem Specifications/Application Functions/SF048A Torque Sensor LOA)' '#SF048A_61' 'true' 'REQ:  SF048A_61' '' } %GIDa_610282b6_286d_46e8_ae0a_31cb5cf47100"  Value=TqLoaDrvrTqNom
  Dead Zone Dynamic : simulink/Discontinuities/Dead Zone Dynamic  RequirementInfo="{'linktype_rmi_doors' '0000ba57 (/E-STEER Core/SubSystem Specifications/Application Functions/SF048A Torque Sensor LOA)' '#SF048A_61' 'true' 'REQ:  SF048A_61' '' } %GIDa_0b0162c1_90dd_45cc_be08_2ef0ee1b704d"
  FixdToFloat_f32_u1 : FixdToFloat/FixdToFloat_f32_u16  RequirementInfo="{'linktype_rmi_doors' '0000ba57 (/E-STEER Core/SubSystem Specifications/Application Functions/SF048A Torque Sensor LOA)' '#SF048A_62' 'true' 'REQ:  SF048A_62' '' } %GIDa_471d00a5_554b_470b_92a0_c209afda8a45"  Param1=12
  FixdToFloat_f32_u16 : FixdToFloat/FixdToFloat_f32_u16  RequirementInfo="{'linktype_rmi_doors' '0000ba57 (/E-STEER Core/SubSystem Specifications/Application Functions/SF048A Torque Sensor LOA)' '#SF048A_60' 'true' 'REQ:  SF048A_60' '' } %GIDa_35ba53a0_e0df_4535_ac1b_211d8cd680e9"  Param1=12
  FloatToFixd_u16_f1 : FloatToFixd/FloatToFixd_u16_f32  RequirementInfo="{'linktype_rmi_doors' '0000ba57 (/E-STEER Core/SubSystem Specifications/Application Functions/SF048A Torque Sensor LOA)' '#SF048A_62' 'true' 'REQ:  SF048A_62' '' } %GIDa_f2fc8a6a_452a_4515_b2d0_a103bc25534e"  Param1=6
  FloatToFixd_u16_f32 : FloatToFixd/FloatToFixd_u16_f32  RequirementInfo="{'linktype_rmi_doors' '0000ba57 (/E-STEER Core/SubSystem Specifications/Application Functions/SF048A Torque Sensor LOA)' '#SF048A_60' 'true' 'REQ:  SF048A_60' '' } %GIDa_35ba7bf2_2c29_46ec_970f_0fba8b58d772"  Param1=6
  LimDyn_f32 : NxtrLim/LimDyn_f32  RequirementInfo="{'linktype_rmi_doors' '0000ba57 (/E-STEER Core/SubSystem Specifications/Application Functions/SF048A Torque Sensor LOA)' '#SF048A_62' 'true' 'REQ:  SF048A_62' '' } %GIDa_b10b9730_f85d_4f89_a039_35eadef39e69"
  LnrIntrpn_u16_u16VariXu16VariY : LnrIntrpn/LnrIntrpn_u16_u16VariXu16VariY  RequirementInfo="{'linktype_rmi_doors' '0000ba57 (/E-STEER Core/SubSystem Specifications/Application Functions/SF048A Torque Sensor LOA)' '#SF048A_60' 'true' 'REQ:  SF048A_60' '' } %GIDa_61d2028c_2510_4991_98e5_e31201526ccd"  XTbl=TqLoaVehSpdX  YTbl=TqLoaVehLatAGainY
      settings: AttributesFormatString=Lnr ( u16VariX , u16VariY )
  LnrIntrpn_u16_u16VariXu16VariY1 : LnrIntrpn/LnrIntrpn_u16_u16VariXu16VariY  RequirementInfo="{'linktype_rmi_doors' '0000ba57 (/E-STEER Core/SubSystem Specifications/Application Functions/SF048A Torque Sensor LOA)' '#SF048A_62' 'true' 'REQ:  SF048A_62' '' } %GIDa_c1283f76_7656_47b8_ba28_e533bebac01e"  XTbl=TqLoaVehSpdX  YTbl=TqLoaTqCmdLimY
      settings: AttributesFormatString=Lnr ( u16VariX , u16VariY )
  Product2 : Product  RequirementInfo="{'linktype_rmi_doors' '0000ba57 (/E-STEER Core/SubSystem Specifications/Application Functions/SF048A Torque Sensor LOA)' '#SF048A_60' 'true' 'REQ:  SF048A_60' '' } %GIDa_7f328ac8_7b38_4e97_a06f_2fbc47d0a532"  RndMeth=Zero
  Subsystem4 : Subsystem  Description=|  mask(Copyright Information){none=on}
      | Copyright info block.                                               
      |                                                                     
      | Place copyright information at the top of every subsystem in design.
      mask prompts: none "No parameters"
      mask help: Place copyright information at the top of every subsystem in design.
      mask Display:
      | NxtrConf = 'Nexteer Confidential';
      | 
      | sys = bdroot; %handle for the current model ("system")
      | first = get_param(sys,'Created');
      | first = first(end-3:end);  %year is last four digits
      | 
      | last = get_param(sys,'LastModifiedDate');
      | if isempty(last)
      |     last = datestr(now,'yyyy');
      | else
      |     last = last(end-3:end);
      | end
      | 
      | if strcmp(first,last)
      |     fprintf('%s\nCopyright  %s Nexteer',NxtrConf,first);
      | else
      |     fprintf('%s\n%s%s-%s Nexteer',NxtrConf,char(169),first,last);
      | end
  Unary Minus : UnaryMinus  RequirementInfo="{'linktype_rmi_doors' '0000ba57 (/E-STEER Core/SubSystem Specifications/Application Functions/SF048A Torque Sensor LOA)' '#SF048A_62' 'true' 'REQ:  SF048A_62' '' } %GIDa_c948c929_e4d7_4695_ad51_bd47ebffc272"
  Unary Minus1 : UnaryMinus  RequirementInfo="{'linktype_rmi_doors' '0000ba57 (/E-STEER Core/SubSystem Specifications/Application Functions/SF048A Torque Sensor LOA)' '#SF048A_61' 'true' 'REQ:  SF048A_61' '' } %GIDa_9cc29c6f_3dae_403b_8ec7_ffa931e58ced"
  TempMtrTrqCmd_MtrNm : Outport  RequirementInfo="{'linktype_rmi_doors' '0000ba57 (/E-STEER Core/SubSystem Specifications/Application Functions/SF048A Torque Sensor LOA)' '#SF048A_62' 'true' 'REQ:  SF048A_62' '' } %GIDa_e6eb04c0_f61e_43bf_b441_8264a0403478"
  wires:
  [Cmd] -> LimDyn_f32/1
  Dead Zone Dynamic/1 -> [Cmd]
  LimDyn_f32/1 -> TempMtrTrqCmd_MtrNm/1
  LnrIntrpn_u16_u16VariXu16VariY1/1 -> FixdToFloat_f32_u1/1
  Unary Minus/1 -> LimDyn_f32/2
  Product2/1 -> Dead Zone Dynamic/2
  VehSpd_kph/1 -> FloatToFixd_u16_f1/1, FloatToFixd_u16_f32/1
  LatAccEst_g/1 -> Product2/1
  LnrIntrpn_u16_u16VariXu16VariY/1 -> FixdToFloat_f32_u16/1
  FloatToFixd_u16_f32/1 -> LnrIntrpn_u16_u16VariXu16VariY/1
  FixdToFloat_f32_u16/1 -> Product2/2
  FixdToFloat_f32_u1/1 -> Unary Minus/1, LimDyn_f32/3
  FloatToFixd_u16_f1/1 -> LnrIntrpn_u16_u16VariXu16VariY1/1
  Constant/1 -> Unary Minus1/1, Dead Zone Dynamic/1
  Unary Minus1/1 -> Dead Zone Dynamic/3

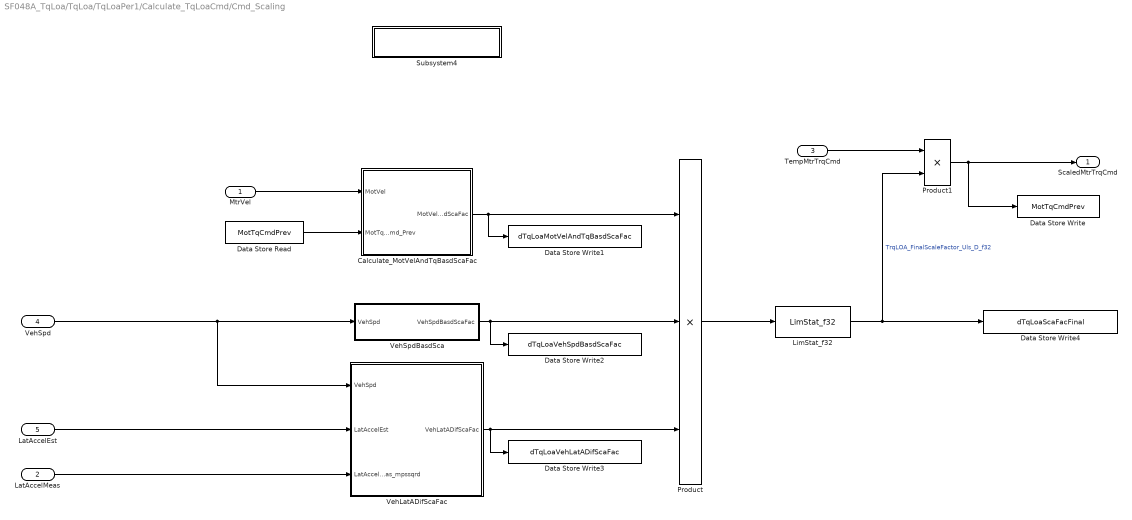
== system SF048A_TqLoa/TqLoa/TqLoaPer1/Calculate_TqLoaCmd/Cmd_Scaling ==
  MtrVel : Inport
  LatAccelMeas : Inport  Port=2
  TempMtrTrqCmd : Inport  RequirementInfo="{'linktype_rmi_doors' '0000ba57 (/E-STEER Core/SubSystem Specifications/Application Functions/SF048A Torque Sensor LOA)' '#SF048A_82' 'true' 'REQ:  SF048A_82' '' } %GIDa_98c41483_329c_4e2a_abde_3a0991d67c86"  Port=3
  VehSpd : Inport  Port=4
  LatAccelEst : Inport  Port=5
  Calculate_MotVelAndTqBasdScaFac : Subsystem
  Data Store Read : DataStoreRead  DataStoreName=MotTqCmdPrev
  Data Store Write : DataStoreWrite  DataStoreName=MotTqCmdPrev
  Data Store Write1 : DataStoreWrite  DataStoreName=dTqLoaMotVelAndTqBasdScaFac
  Data Store Write2 : DataStoreWrite  DataStoreName=dTqLoaVehSpdBasdScaFac
  Data Store Write3 : DataStoreWrite  DataStoreName=dTqLoaVehLatADifScaFac
  Data Store Write4 : DataStoreWrite  DataStoreName=dTqLoaScaFacFinal
  LimStat_f32 : NxtrLim/LimStat_f32  LoLim=MOTTQSCAFACMIN_ULS_F32  HiLim=MOTTQSCAFACMAX_ULS_F32
      settings: AttributesFormatString=|
      | Low Limit: %<LoLim>
      | High Limit:%<HiLim>
  Product : Product  RequirementInfo="{'linktype_rmi_doors' '0000ba57 (/E-STEER Core/SubSystem Specifications/Application Functions/SF048A Torque Sensor LOA)' '#SF048A_73' 'true' 'REQ:  SF048A_73' '' ; 'linktype_rmi_doors' '0000ba57 (/E-STEER Core/SubSystem Specifications/Application Functions/SF048A Torque Sensor LOA)' '#SF048A_79' 'true' 'REQ:  SF048A_79' '' ; 'linktype_rmi_doors' '0000ba57 (/E-STEER Core/SubSystem Specifications/Application Functions/SF048A Torque Sensor LOA)' '#SF048A_81' 'true' 'REQ:  SF048A_81' '' } %GIDa_aa34a325_600c_499d_92bf_a7c7dca47e23"  Inputs=3  RndMeth=Zero
  Product1 : Product  RequirementInfo="{'linktype_rmi_doors' '0000ba57 (/E-STEER Core/SubSystem Specifications/Application Functions/SF048A Torque Sensor LOA)' '#SF048A_82' 'true' 'REQ:  SF048A_82' '' } %GIDa_3b01ad78_19c8_4d10_9d8e_0bfb0c6ed526"  RndMeth=Zero
  Subsystem4 : Subsystem  Description=|  mask(Copyright Information){none=on}
      | Copyright info block.                                               
      |                                                                     
      | Place copyright information at the top of every subsystem in design.
      mask prompts: none "No parameters"
      mask help: Place copyright information at the top of every subsystem in design.
      mask Display:
      | NxtrConf = 'Nexteer Confidential';
      | 
      | sys = bdroot; %handle for the current model ("system")
      | first = get_param(sys,'Created');
      | first = first(end-3:end);  %year is last four digits
      | 
      | last = get_param(sys,'LastModifiedDate');
      | if isempty(last)
      |     last = datestr(now,'yyyy');
      | else
      |     last = last(end-3:end);
      | end
      | 
      | if strcmp(first,last)
      |     fprintf('%s\nCopyright  %s Nexteer',NxtrConf,first);
      | else
      |     fprintf('%s\n%s%s-%s Nexteer',NxtrConf,char(169),first,last);
      | end
  VehLatADifScaFac : Subsystem  RequirementInfo="{'linktype_rmi_doors' '0000ba57 (/E-STEER Core/SubSystem Specifications/Application Functions/SF048A Torque Sensor LOA)' '#SF048A_76' 'true' 'REQ:  SF048A_76' '' } %GIDa_acc9be4d_992e_4791_9272_cb55c4e25398"
  VehSpdBasdSca : Subsystem
  ScaledMtrTrqCmd : Outport  RequirementInfo="{'linktype_rmi_doors' '0000ba57 (/E-STEER Core/SubSystem Specifications/Application Functions/SF048A Torque Sensor LOA)' '#SF048A_82' 'true' 'REQ:  SF048A_82' '' } %GIDa_d1f2059e_3e08_4894_9b5f_11b5ebe3ee6a"
  wires:
  Data Store Read/1 -> Calculate_MotVelAndTqBasdScaFac/2(MotTqCmd_Prev)
  VehLatADifScaFac/1(VehLatADifScaFac) -> Data Store Write3/1, Product/3
  VehSpdBasdSca/1(VehSpdBasdScaFac) -> Data Store Write2/1, Product/2
  Calculate_MotVelAndTqBasdScaFac/1(MotVelAndTqBasdScaFac) -> Data Store Write1/1, Product/1
  LimStat_f32/1 -> Data Store Write4/1, Product1/2  "TrqLOA_FinalScaleFactor_Uls_D_f32"
  Product1/1 -> Data Store Write/1, ScaledMtrTrqCmd/1
  TempMtrTrqCmd/1 -> Product1/1
  Product/1 -> LimStat_f32/1
  MtrVel/1 -> Calculate_MotVelAndTqBasdScaFac/1(MotVel)
  LatAccelEst/1 -> VehLatADifScaFac/2(LatAccelEst)
  VehSpd/1 -> VehSpdBasdSca/1(VehSpd), VehLatADifScaFac/1(VehSpd)
  LatAccelMeas/1 -> VehLatADifScaFac/3(LatAccelMeas_mpssqrd)

== system SF048A_TqLoa/TqLoa/TqLoaPer1/Calculate_TqLoaCmd/Subsystem4 ==

== system SF048A_TqLoa/TqLoa/TqLoaPer1/Estimate Lateral Acceleration/Subsystem4 ==

== system SF048A_TqLoa/TqLoa/TqLoaPer1/ValidityCheck/If Action Subsystem ==
  In1 : Inport
  Action Port : ActionPort  ActionType=then
  Subsystem4 : Subsystem  Description=|  mask(Copyright Information){none=on}
      | Copyright info block.                                               
      |                                                                     
      | Place copyright information at the top of every subsystem in design.
      mask prompts: none "No parameters"
      mask help: Place copyright information at the top of every subsystem in design.
      mask Display:
      | NxtrConf = 'Nexteer Confidential';
      | 
      | sys = bdroot; %handle for the current model ("system")
      | first = get_param(sys,'Created');
      | first = first(end-3:end);  %year is last four digits
      | 
      | last = get_param(sys,'LastModifiedDate');
      | if isempty(last)
      |     last = datestr(now,'yyyy');
      | else
      |     last = last(end-3:end);
      | end
      | 
      | if strcmp(first,last)
      |     fprintf('%s\nCopyright  %s Nexteer',NxtrConf,first);
      | else
      |     fprintf('%s\n%s%s-%s Nexteer',NxtrConf,char(169),first,last);
      | end
  Out1 : Outport
  wires:
  In1/1 -> Out1/1

== system SF048A_TqLoa/TqLoa/TqLoaPer1/ValidityCheck/If Action Subsystem1 ==
  In1 : Inport
  Action Port : ActionPort  ActionType=else
  Subsystem4 : Subsystem  Description=|  mask(Copyright Information){none=on}
      | Copyright info block.                                               
      |                                                                     
      | Place copyright information at the top of every subsystem in design.
      mask prompts: none "No parameters"
      mask help: Place copyright information at the top of every subsystem in design.
      mask Display:
      | NxtrConf = 'Nexteer Confidential';
      | 
      | sys = bdroot; %handle for the current model ("system")
      | first = get_param(sys,'Created');
      | first = first(end-3:end);  %year is last four digits
      | 
      | last = get_param(sys,'LastModifiedDate');
      | if isempty(last)
      |     last = datestr(now,'yyyy');
      | else
      |     last = last(end-3:end);
      | end
      | 
      | if strcmp(first,last)
      |     fprintf('%s\nCopyright  %s Nexteer',NxtrConf,first);
      | else
      |     fprintf('%s\n%s%s-%s Nexteer',NxtrConf,char(169),first,last);
      | end
  Out1 : Outport
  wires:
  In1/1 -> Out1/1

== system SF048A_TqLoa/TqLoa/TqLoaPer1/ValidityCheck/Subsystem4 ==

== system SF048A_TqLoa/TqLoa/TqLoaPer1/Calculate_TqLoaCmd/Calculate_TqCmd/Subsystem4 ==

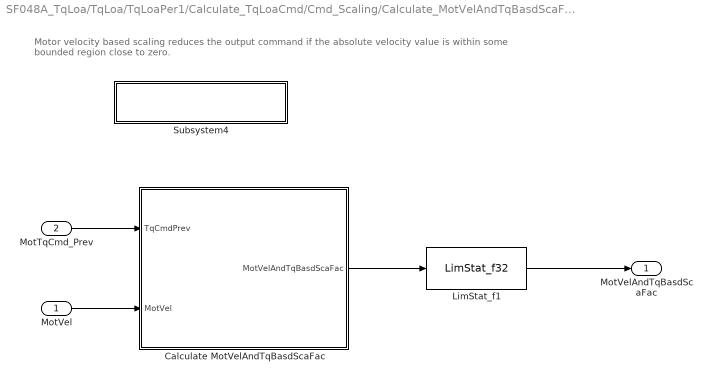
== system SF048A_TqLoa/TqLoa/TqLoaPer1/Calculate_TqLoaCmd/Cmd_Scaling/Calculate_MotVelAndTqBasdScaFac ==
  note: Motor velocity based scaling reduces the output command if the
      | absolute velocity value is within some bounded region close to zero.
  MotVel : Inport  RequirementInfo="{'linktype_rmi_doors' '0000ba57 (/E-STEER Core/SubSystem Specifications/Application Functions/SF048A Torque Sensor LOA)' '#SF048A_65' 'true' 'REQ:  SF048A_65' '' } %GIDa_b89109a2_3e96_4899_bf63_f3148ee9ce3a"
  MotTqCmd_Prev : Inport  RequirementInfo="{'linktype_rmi_doors' '0000ba57 (/E-STEER Core/SubSystem Specifications/Application Functions/SF048A Torque Sensor LOA)' '#SF048A_65' 'true' 'REQ:  SF048A_65' '' } %GIDa_4539cd14_2fc8_456f_9a60_09f18f0a05bf"  Port=2
  Calculate MotVelAndTqBasdScaFac : Subsystem  RequirementInfo="{'linktype_rmi_doors' '0000ba57 (/E-STEER Core/SubSystem Specifications/Application Functions/SF048A Torque Sensor LOA)' '#SF048A_65' 'true' 'REQ:  SF048A_65' '' } %GIDa_d831dac1_a3f6_4788_8baa_6028cb9a2476"
  LimStat_f1 : NxtrLim/LimStat_f32  RequirementInfo="{'linktype_rmi_doors' '0000ba57 (/E-STEER Core/SubSystem Specifications/Application Functions/SF048A Torque Sensor LOA)' '#SF048A_69' 'true' 'REQ:  SF048A_69' '' } %GIDa_18f0599a_4299_457d_8907_6592b3160107"  LoLim=MOTTQSCAFACMIN_ULS_F32  HiLim=MOTTQSCAFACMAX_ULS_F32
      settings: AttributesFormatString=|
      | Low Limit: %<LoLim>
      | High Limit:%<HiLim>
  Subsystem4 : Subsystem  Description=|  mask(Copyright Information){none=on}
      | Copyright info block.                                               
      |                                                                     
      | Place copyright information at the top of every subsystem in design.
      mask prompts: none "No parameters"
      mask help: Place copyright information at the top of every subsystem in design.
      mask Display:
      | NxtrConf = 'Nexteer Confidential';
      | 
      | sys = bdroot; %handle for the current model ("system")
      | first = get_param(sys,'Created');
      | first = first(end-3:end);  %year is last four digits
      | 
      | last = get_param(sys,'LastModifiedDate');
      | if isempty(last)
      |     last = datestr(now,'yyyy');
      | else
      |     last = last(end-3:end);
      | end
      | 
      | if strcmp(first,last)
      |     fprintf('%s\nCopyright  %s Nexteer',NxtrConf,first);
      | else
      |     fprintf('%s\n%s%s-%s Nexteer',NxtrConf,char(169),first,last);
      | end
  MotVelAndTqBasdScaFac : Outport
  wires:
  Calculate MotVelAndTqBasdScaFac/1(MotVelAndTqBasdScaFac) -> LimStat_f1/1
  MotVel/1 -> Calculate MotVelAndTqBasdScaFac/2(MotVel)
  MotTqCmd_Prev/1 -> Calculate MotVelAndTqBasdScaFac/1(TqCmdPrev)
  LimStat_f1/1 -> MotVelAndTqBasdScaFac/1

== system SF048A_TqLoa/TqLoa/TqLoaPer1/Calculate_TqLoaCmd/Cmd_Scaling/Subsystem4 ==
